simulink model "SMA_displacementIn_PC2_6"  (R2018a)
settings: Solver=ode15s  StartTime=0.0  StopTime=100  RelTol=1e-8  AbsTol=1e-8  EnableMultiTasking=on
values from neighbouring files (symbols this model uses):
  param_b = 10    [plot_task_6.m]
  param_con_I = param_con_P/(0.85*0.9)    (= 1.29411764706)    [plot_task_6.m]
  param_con_P = 0.45*2.2    (= 0.99)    [plot_task_6.m]
  param_factor = 0.0137    [plot_task_6.m]
  param_J = params_PC2.alpha * 2 * pi * params_PC2.r0 * params_PC2.L0 * param_N * params_PC2.delta_T    [plot_task_6.m]
  param_J0_yin = 0.7845    [plot_task_6.m]
  param_k = 500    [plot_task_6.m]
  param_lin_a0 = 0.092    [plot_task_6.m]
  param_lin_a1 = - 7/675    (= -0.0103703703704)    [plot_task_6.m]
  param_lin_q_max = 0.014    [plot_task_6.m]
  param_m = 0.3    [plot_task_6.m]
  param_N = 20    [plot_task_6.m]
undefined symbols (not defined in the file or in its folder): params_PC2
libraries: simulink x1
settings Model: Creator=Gianluca  LastModifiedBy=tim
settings SolverCC: AutoScaleAbsTol=off
settings DataIOCC: LimitDataPoints=on  SaveFormat=Array
settings OptimizationCC: LifeSpan=inf
settings DebuggingCC: UnderspecifiedInitializationDetection=Classic  MergeDetectMultiDrivingBlocksExec=none  SolverPrmCheckMsg=warning  StateNameClashWarn=warning  SFUnexpectedBacktrackingDiag=warning  SFNoUnconditionalDefaultTransitionDiag=warning  SFExecutionAtInitializationDiag=none
settings HardwareCC: ProdBitPerPointer=32  ProdBitPerSizeT=32  ProdBitPerPtrDiffT=32  ProdLargestAtomicFloat=None  ProdIntDivRoundTo=Undefined  ProdEndianess=Unspecified  ProdWordSize=32  ProdHWDeviceType=32-bit Generic
settings ModelReferenceCC: PropagateSignalLabelsOutOfModel=off
settings CodeAppCC: StateflowObjectComments=on
settings GRTTargetCC: TargetLangStandard=C89/C90 (ANSI)  GeneratePreprocessorConditionals=Disable all
settings ConfigComp: CovMetricSettings=dw  CovHtmlReporting=on  CovSaveCumulativeToWorkspaceVar=on  CovSaveSingleToWorkspaceVar=on  CovExternalEMLEnable=off

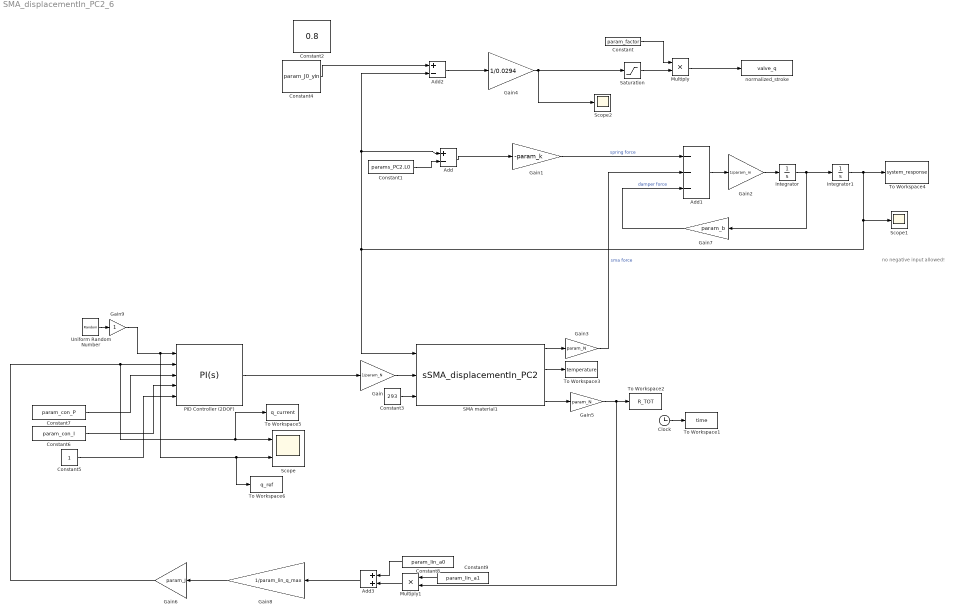
== system SMA_displacementIn_PC2_6 ==
  note: no negative input allowed!
  Add : Sum  Inputs=+-
  Add1 : Sum  Inputs=---
  Add2 : Sum  Inputs=+-
  Add3 : Sum
  Clock : Clock
  Constant : Constant  Value=param_factor
  Constant1 : Constant  Value=params_PC2.L0
  Constant2 : Constant  Value=0.8
  Constant3 : Constant  Value=293
  Constant4 : Constant  Value=param_J0_yin
  Constant5 : Constant
  Constant6 : Constant  Value=param_con_I
  Constant7 : Constant  Value=param_con_P
  Constant8 : Constant  Value=param_lin_a0
  Constant9 : Constant  Value=param_lin_a1
  Gain : Gain  Gain=1/param_N
  Gain1 : Gain  Gain=-param_k
  Gain2 : Gain  Gain=1/param_m
  Gain3 : Gain  Gain=param_N
  Gain4 : Gain  Gain=1/0.0294
  Gain5 : Gain  Gain=param_N
  Gain6 : Gain  Gain=param_J
  Gain7 : Gain  Gain=param_b
  Gain8 : Gain  Gain=1/param_lin_q_max
  Gain9 : Gain
  Integrator : Integrator
  Integrator1 : Integrator  InitialCondition=param_J0_yin
  Multiply : Product
  Multiply1 : Product
  PID Controller (2DOF) : simulink/Continuous/PID Controller (2DOF)  Controller=PI  TimeDomain=Continuous-time  SampleTime=-1  IntegratorMethod=Forward Euler  FilterMethod=Forward Euler  Form=Parallel  UseFilter=on  ControllerParametersSource=external  P=1  I=1  D=0  N=100  b=1  c=1  InitialConditionSource=internal  InitialConditionForIntegrator=0  InitialConditionForFilter=0  ExternalReset=none  LimitOutput=on  UpperSaturationLimit=param_J  LowerSaturationLimit=0  LinearizeAsGain=on  AntiWindupMode=back-calculation  Kb=1  TrackingMode=off  Kt=1  PParamMin=[]  PParamMax=[]  IParamMin=[]  IParamMax=[]  DParamMin=[]  DParamMax=[]  NParamMin=[]  NParamMax=[]  bParamMin=[]  bParamMax=[]  cParamMin=[]  cParamMax=[]  KbParamMin=[]  KbParamMax=[]  KtParamMin=[]  KtParamMax=[]  POutMin=[]  POutMax=[]  IOutMin=[]  IOutMax=[]  DOutMin=[]  DOutMax=[]  NOutMin=[]  NOutMax=[]  bOutMin=[]  bOutMax=[]  cOutMin=[]  cOutMax=[]  KbOutMin=[]  KbOutMax=[]  KtOutMin=[]  KtOutMax=[]  IntegratorOutMin=[]  IntegratorOutMax=[]  FilterOutMin=[]  FilterOutMax=[]  SumOutMin=[]  SumOutMax=[]  Sum1OutMin=[]  Sum1OutMax=[]  Sum2OutMin=[]  Sum2OutMax=[]  Sum3OutMin=[]  Sum3OutMax=[]  SumI1OutMin=[]  SumI1OutMax=[]  SumI2OutMin=[]  SumI2OutMax=[]  SumI3OutMin=[]  SumI3OutMax=[]  SumDOutMin=[]  SumDOutMax=[]  SaturationOutMin=[]  SaturationOutMax=[]  IntegratorContinuousStateAttributes=''  IntegratorStateMustResolveToSignalObject=off  IntegratorRTWStateStorageClass=Auto  FilterContinuousStateAttributes=''  FilterStateMustResolveToSignalObject=off  FilterRTWStateStorageClass=Auto  DifferentiatorICPrevScaledInput=0  DifferentiatorOutMin=[]  DifferentiatorOutMax=[]  FilterDiffOutCoefMin=[]  FilterDiffOutCoefMax=[]  SumDenOutMin=[]  SumDenOutMax=[]  SumNumOutMin=[]  SumNumOutMax=[]  ReciprocalOutMin=[]  ReciprocalOutMax=[]  DivideOutMin=[]  DivideOutMax=[]  TunerSelectOption=Transfer Function Based (PID Tuner App)
  SMA material1 : M-S-Function  FunctionName=sSMA_displacementIn_PC2  Parameters=params_PC2, initConds_PC2
      mask Display:
      | color('black');
      | patch(3*[-1 1 1 -1],1.1*[-1 -1 1 1],[1 1 1]);
      | patch([-1.6 -0.8],[-0.9 0.3],[0 0 0]);
      | patch([-0.8 1.2],[0.3 0.3],[0 0 0]);
      | patch([1.6 0.8],[0.9 -0.3],[0 0 0]);
      | patch([0.8 -1.2],[-0.3 -0.3],[0 0 0]);
      | disp('SMA');
      | 
      | color('blue');
      | port_label('input', 1, 'y [m]','texmode','on');
      | port_label('input', 2, 'J [W]','texmode','on');
      | port_label('input', 3, 'T_E [K]','texmode','on');
      | 
      | color('red');
      | port_label('output', 1, 'F [N]','texmode','on');
      | port_label('output', 2, 'x_+, x_-, x_A [-]','texmode','on');
      | port_label('output', 3, 'T [K]','texmode','on');
      | port_label('output', 4, '\epsilon [-]','texmode','on');
      | port_label('output', 5, '\sigma [Pa]','texmode','on');
      | port_label('output', 6, 'R [\Omega]','texmode','on');
  Saturation : Saturate  UpperLimit=1  LowerLimit=0
  Scope : Scope  NumInputPorts=2
  Scope1 : Scope
  Scope2 : Scope
  To Workspace1 : ToWorkspace  VariableName=time  SampleTime=-1
  To Workspace2 : ToWorkspace  VariableName=R_TOT  SampleTime=-1
  To Workspace3 : ToWorkspace  VariableName=temperature  SampleTime=-1
  To Workspace4 : ToWorkspace  VariableName=system_response  SampleTime=-1
  To Workspace5 : ToWorkspace  VariableName=q_current  SampleTime=-1
  To Workspace6 : ToWorkspace  VariableName=q_ref
  Uniform Random Number : UniformRandomNumber  Minimum=0  Maximum=param_J  Seed=3456789  SampleTime=20
  normalized_stroke : ToWorkspace  VariableName=valve_q  SampleTime=-1
  wires:
  Gain7/1 -> Add1/3  "damper force"
  Integrator/1 -> Integrator1/1, Gain7/1
  Gain3/1 -> Add1/2  "sma force"
  PID Controller (2DOF)/1 -> Gain/1
  Constant3/1 -> SMA material1/3
  SMA material1/1 -> Gain3/1
  SMA material1/3 -> To Workspace3/1
  Gain/1 -> SMA material1/2
  Gain1/1 -> Add1/1  "spring force"
  Add1/1 -> Gain2/1
  Gain2/1 -> Integrator/1
  Gain4/1 -> Saturation/1, Scope2/1
  Add2/1 -> Gain4/1
  Integrator1/1 -> To Workspace4/1, Add/1, Add2/2, SMA material1/1, Scope1/1
  Add/1 -> Gain1/1
  Clock/1 -> To Workspace1/1
  Constant1/1 -> Add/2
  Constant4/1 -> Add2/1
  Constant/1 -> Multiply/1
  Multiply/1 -> normalized_stroke/1
  Saturation/1 -> Multiply/2
  SMA material1/6 -> Gain5/1
  Gain5/1 -> Multiply1/2, To Workspace2/1
  Constant5/1 -> PID Controller (2DOF)/5
  Constant6/1 -> PID Controller (2DOF)/4
  Constant7/1 -> PID Controller (2DOF)/3
  Uniform Random Number/1 -> Gain9/1
  Multiply1/1 -> Add3/2
  Constant8/1 -> Add3/1
  Constant9/1 -> Multiply1/1
  Add3/1 -> Gain8/1
  Gain8/1 -> Gain6/1
  Gain6/1 -> To Workspace5/1, Scope/1, PID Controller (2DOF)/2
  Gain9/1 -> To Workspace6/1, Scope/2, PID Controller (2DOF)/1
